simulink model "CommSys_300_Bus_Area2"  (Simulink 8.0)
settings: Solver=ode45  StartTime=0.0  StopTime=85  RelTol=1e-3
libraries: PiccSIM x86
settings Model: Creator=svenda  LastModifiedBy=svenda

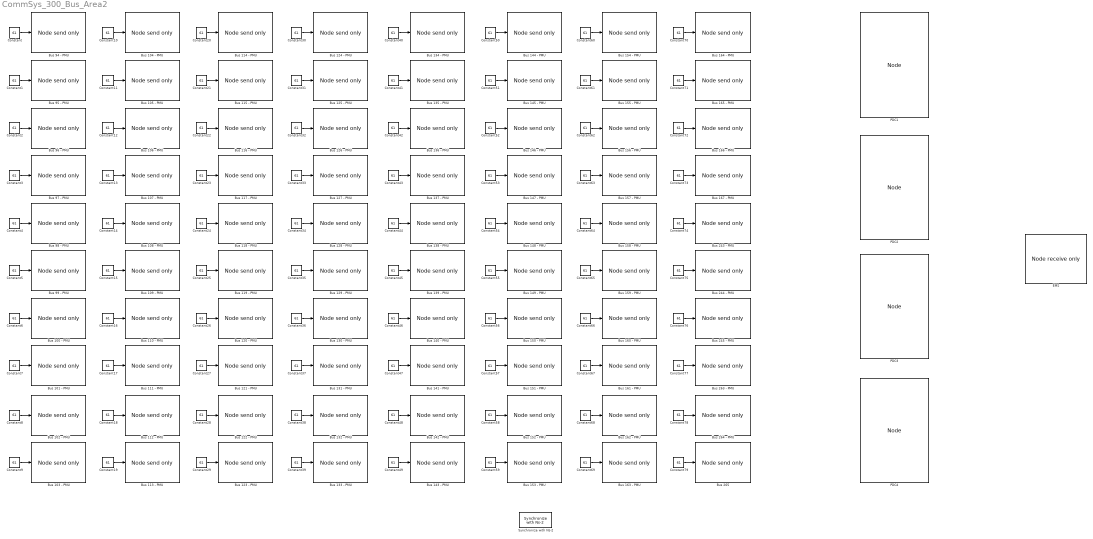
== system CommSys_300_Bus_Area2 ==
  Bus 100 - PMU : PiccSIM/Node send only  ID=6  time_or_seq=Timestamp  sendSchedule=Fixed sampling time  h=0.02  duty_cycle=1  sendEnable=off  pTypesSend=[16]  sendDataStructure={{'double'}}  externalID=off  sendID={[80]}  coordinates=[0, 0]  IP=NS2_IP
  Bus 101 - PMU : PiccSIM/Node send only  ID=7  time_or_seq=Timestamp  sendSchedule=Fixed sampling time  h=0.02  duty_cycle=1  sendEnable=off  pTypesSend=[17]  sendDataStructure={{'double'}}  externalID=off  sendID={[80]}  coordinates=[0, 0]  IP=NS2_IP
  Bus 102 - PMU : PiccSIM/Node send only  ID=8  time_or_seq=Timestamp  sendSchedule=Fixed sampling time  h=0.02  duty_cycle=1  sendEnable=off  pTypesSend=[18]  sendDataStructure={{'double'}}  externalID=off  sendID={[80]}  coordinates=[0, 0]  IP=NS2_IP
  Bus 103 - PMU : PiccSIM/Node send only  ID=9  time_or_seq=Timestamp  sendSchedule=Fixed sampling time  h=0.02  duty_cycle=1  sendEnable=off  pTypesSend=[19]  sendDataStructure={{'double'}}  externalID=off  sendID={[80]}  coordinates=[0, 0]  IP=NS2_IP
  Bus 104 - PMU : PiccSIM/Node send only  ID=10  time_or_seq=Timestamp  sendSchedule=Fixed sampling time  h=0.02  duty_cycle=1  sendEnable=off  pTypesSend=[110]  sendDataStructure={{'double'}}  externalID=off  sendID={[80]}  coordinates=[0, 0]  IP=NS2_IP
  Bus 105 - PMU : PiccSIM/Node send only  ID=11  time_or_seq=Timestamp  sendSchedule=Fixed sampling time  h=0.02  duty_cycle=1  sendEnable=off  pTypesSend=[111]  sendDataStructure={{'double'}}  externalID=off  sendID={[80]}  coordinates=[0, 0]  IP=NS2_IP
  Bus 106 - PMU : PiccSIM/Node send only  ID=12  time_or_seq=Timestamp  sendSchedule=Fixed sampling time  h=0.02  duty_cycle=1  sendEnable=off  pTypesSend=[112]  sendDataStructure={{'double'}}  externalID=off  sendID={[80]}  coordinates=[0, 0]  IP=NS2_IP
  Bus 107 - PMU : PiccSIM/Node send only  ID=13  time_or_seq=Timestamp  sendSchedule=Fixed sampling time  h=0.02  duty_cycle=1  sendEnable=off  pTypesSend=[113]  sendDataStructure={{'double'}}  externalID=off  sendID={[80]}  coordinates=[0, 0]  IP=NS2_IP
  Bus 108 - PMU : PiccSIM/Node send only  ID=14  time_or_seq=Timestamp  sendSchedule=Fixed sampling time  h=0.02  duty_cycle=1  sendEnable=off  pTypesSend=[114]  sendDataStructure={{'double'}}  externalID=off  sendID={[80]}  coordinates=[0, 0]  IP=NS2_IP
  Bus 109 - PMU : PiccSIM/Node send only  ID=15  time_or_seq=Timestamp  sendSchedule=Fixed sampling time  h=0.02  duty_cycle=1  sendEnable=off  pTypesSend=[115]  sendDataStructure={{'double'}}  externalID=off  sendID={[80]}  coordinates=[0, 0]  IP=NS2_IP
  Bus 110 - PMU : PiccSIM/Node send only  ID=16  time_or_seq=Timestamp  sendSchedule=Fixed sampling time  h=0.02  duty_cycle=1  sendEnable=off  pTypesSend=[116]  sendDataStructure={{'double'}}  externalID=off  sendID={[80]}  coordinates=[0, 0]  IP=NS2_IP
  Bus 111 - PMU : PiccSIM/Node send only  ID=17  time_or_seq=Timestamp  sendSchedule=Fixed sampling time  h=0.02  duty_cycle=1  sendEnable=off  pTypesSend=[117]  sendDataStructure={{'double'}}  externalID=off  sendID={[80]}  coordinates=[0, 0]  IP=NS2_IP
  Bus 112 - PMU : PiccSIM/Node send only  ID=18  time_or_seq=Timestamp  sendSchedule=Fixed sampling time  h=0.02  duty_cycle=1  sendEnable=off  pTypesSend=[118]  sendDataStructure={{'double'}}  externalID=off  sendID={[80]}  coordinates=[0, 0]  IP=NS2_IP
  Bus 113 - PMU : PiccSIM/Node send only  ID=19  time_or_seq=Timestamp  sendSchedule=Fixed sampling time  h=0.02  duty_cycle=1  sendEnable=off  pTypesSend=[119]  sendDataStructure={{'double'}}  externalID=off  sendID={[80]}  coordinates=[0, 0]  IP=NS2_IP
  Bus 114 - PMU : PiccSIM/Node send only  ID=20  time_or_seq=Timestamp  sendSchedule=Fixed sampling time  h=0.02  duty_cycle=1  sendEnable=off  pTypesSend=[120]  sendDataStructure={{'double'}}  externalID=off  sendID={[81]}  coordinates=[0, 0]  IP=NS2_IP
  Bus 115 - PMU : PiccSIM/Node send only  ID=21  time_or_seq=Timestamp  sendSchedule=Fixed sampling time  h=0.02  duty_cycle=1  sendEnable=off  pTypesSend=[121]  sendDataStructure={{'double'}}  externalID=off  sendID={[81]}  coordinates=[0, 0]  IP=NS2_IP
  Bus 116 - PMU : PiccSIM/Node send only  ID=22  time_or_seq=Timestamp  sendSchedule=Fixed sampling time  h=0.02  duty_cycle=1  sendEnable=off  pTypesSend=[122]  sendDataStructure={{'double'}}  externalID=off  sendID={[81]}  coordinates=[0, 0]  IP=NS2_IP
  Bus 117 - PMU : PiccSIM/Node send only  ID=23  time_or_seq=Timestamp  sendSchedule=Fixed sampling time  h=0.02  duty_cycle=1  sendEnable=off  pTypesSend=[123]  sendDataStructure={{'double'}}  externalID=off  sendID={[81]}  coordinates=[0, 0]  IP=NS2_IP
  Bus 118 - PMU : PiccSIM/Node send only  ID=24  time_or_seq=Timestamp  sendSchedule=Fixed sampling time  h=0.02  duty_cycle=1  sendEnable=off  pTypesSend=[124]  sendDataStructure={{'double'}}  externalID=off  sendID={[81]}  coordinates=[0, 0]  IP=NS2_IP
  Bus 119 - PMU : PiccSIM/Node send only  ID=25  time_or_seq=Timestamp  sendSchedule=Fixed sampling time  h=0.02  duty_cycle=1  sendEnable=off  pTypesSend=[125]  sendDataStructure={{'double'}}  externalID=off  sendID={[81]}  coordinates=[0, 0]  IP=NS2_IP
  Bus 120 - PMU : PiccSIM/Node send only  ID=26  time_or_seq=Timestamp  sendSchedule=Fixed sampling time  h=0.02  duty_cycle=1  sendEnable=off  pTypesSend=[126]  sendDataStructure={{'double'}}  externalID=off  sendID={[81]}  coordinates=[0, 0]  IP=NS2_IP
  Bus 121 - PMU : PiccSIM/Node send only  ID=27  time_or_seq=Timestamp  sendSchedule=Fixed sampling time  h=0.02  duty_cycle=1  sendEnable=off  pTypesSend=[127]  sendDataStructure={{'double'}}  externalID=off  sendID={[81]}  coordinates=[0, 0]  IP=NS2_IP
  Bus 122 - PMU : PiccSIM/Node send only  ID=28  time_or_seq=Timestamp  sendSchedule=Fixed sampling time  h=0.02  duty_cycle=1  sendEnable=off  pTypesSend=[128]  sendDataStructure={{'double'}}  externalID=off  sendID={[81]}  coordinates=[0, 0]  IP=NS2_IP
  Bus 123 - PMU : PiccSIM/Node send only  ID=29  time_or_seq=Timestamp  sendSchedule=Fixed sampling time  h=0.02  duty_cycle=1  sendEnable=off  pTypesSend=[129]  sendDataStructure={{'double'}}  externalID=off  sendID={[81]}  coordinates=[0, 0]  IP=NS2_IP
  Bus 124 - PMU : PiccSIM/Node send only  ID=30  time_or_seq=Timestamp  sendSchedule=Fixed sampling time  h=0.02  duty_cycle=1  sendEnable=off  pTypesSend=[130]  sendDataStructure={{'double'}}  externalID=off  sendID={[81]}  coordinates=[0, 0]  IP=NS2_IP
  Bus 125 - PMU : PiccSIM/Node send only  ID=31  time_or_seq=Timestamp  sendSchedule=Fixed sampling time  h=0.02  duty_cycle=1  sendEnable=off  pTypesSend=[131]  sendDataStructure={{'double'}}  externalID=off  sendID={[81]}  coordinates=[0, 0]  IP=NS2_IP
  Bus 126 - PMU : PiccSIM/Node send only  ID=32  time_or_seq=Timestamp  sendSchedule=Fixed sampling time  h=0.02  duty_cycle=1  sendEnable=off  pTypesSend=[132]  sendDataStructure={{'double'}}  externalID=off  sendID={[81]}  coordinates=[0, 0]  IP=NS2_IP
  Bus 127 - PMU : PiccSIM/Node send only  ID=33  time_or_seq=Timestamp  sendSchedule=Fixed sampling time  h=0.02  duty_cycle=1  sendEnable=off  pTypesSend=[133]  sendDataStructure={{'double'}}  externalID=off  sendID={[81]}  coordinates=[0, 0]  IP=NS2_IP
  Bus 128 - PMU : PiccSIM/Node send only  ID=34  time_or_seq=Timestamp  sendSchedule=Fixed sampling time  h=0.02  duty_cycle=1  sendEnable=off  pTypesSend=[134]  sendDataStructure={{'double'}}  externalID=off  sendID={[81]}  coordinates=[0, 0]  IP=NS2_IP
  Bus 129 - PMU : PiccSIM/Node send only  ID=35  time_or_seq=Timestamp  sendSchedule=Fixed sampling time  h=0.02  duty_cycle=1  sendEnable=off  pTypesSend=[135]  sendDataStructure={{'double'}}  externalID=off  sendID={[81]}  coordinates=[0, 0]  IP=NS2_IP
  Bus 130 - PMU : PiccSIM/Node send only  ID=36  time_or_seq=Timestamp  sendSchedule=Fixed sampling time  h=0.02  duty_cycle=1  sendEnable=off  pTypesSend=[136]  sendDataStructure={{'double'}}  externalID=off  sendID={[81]}  coordinates=[0, 0]  IP=NS2_IP
  Bus 131 - PMU : PiccSIM/Node send only  ID=37  time_or_seq=Timestamp  sendSchedule=Fixed sampling time  h=0.02  duty_cycle=1  sendEnable=off  pTypesSend=[137]  sendDataStructure={{'double'}}  externalID=off  sendID={[81]}  coordinates=[0, 0]  IP=NS2_IP
  Bus 132 - PMU : PiccSIM/Node send only  ID=38  time_or_seq=Timestamp  sendSchedule=Fixed sampling time  h=0.02  duty_cycle=1  sendEnable=off  pTypesSend=[138]  sendDataStructure={{'double'}}  externalID=off  sendID={[81]}  coordinates=[0, 0]  IP=NS2_IP
  Bus 133 - PMU : PiccSIM/Node send only  ID=39  time_or_seq=Timestamp  sendSchedule=Fixed sampling time  h=0.02  duty_cycle=1  sendEnable=off  pTypesSend=[139]  sendDataStructure={{'double'}}  externalID=off  sendID={[81]}  coordinates=[0, 0]  IP=NS2_IP
  Bus 134 - PMU : PiccSIM/Node send only  ID=40  time_or_seq=Timestamp  sendSchedule=Fixed sampling time  h=0.02  duty_cycle=1  sendEnable=off  pTypesSend=[140]  sendDataStructure={{'double'}}  externalID=off  sendID={[82]}  coordinates=[0, 0]  IP=NS2_IP
  Bus 135 - PMU : PiccSIM/Node send only  ID=41  time_or_seq=Timestamp  sendSchedule=Fixed sampling time  h=0.02  duty_cycle=1  sendEnable=off  pTypesSend=[141]  sendDataStructure={{'double'}}  externalID=off  sendID={[82]}  coordinates=[0, 0]  IP=NS2_IP
  Bus 136 - PMU : PiccSIM/Node send only  ID=42  time_or_seq=Timestamp  sendSchedule=Fixed sampling time  h=0.02  duty_cycle=1  sendEnable=off  pTypesSend=[142]  sendDataStructure={{'double'}}  externalID=off  sendID={[82]}  coordinates=[0, 0]  IP=NS2_IP
  Bus 137 - PMU : PiccSIM/Node send only  ID=43  time_or_seq=Timestamp  sendSchedule=Fixed sampling time  h=0.02  duty_cycle=1  sendEnable=off  pTypesSend=[143]  sendDataStructure={{'double'}}  externalID=off  sendID={[82]}  coordinates=[0, 0]  IP=NS2_IP
  Bus 138 - PMU : PiccSIM/Node send only  ID=44  time_or_seq=Timestamp  sendSchedule=Fixed sampling time  h=0.02  duty_cycle=1  sendEnable=off  pTypesSend=[144]  sendDataStructure={{'double'}}  externalID=off  sendID={[82]}  coordinates=[0, 0]  IP=NS2_IP
  Bus 139 - PMU : PiccSIM/Node send only  ID=45  time_or_seq=Timestamp  sendSchedule=Fixed sampling time  h=0.02  duty_cycle=1  sendEnable=off  pTypesSend=[145]  sendDataStructure={{'double'}}  externalID=off  sendID={[82]}  coordinates=[0, 0]  IP=NS2_IP
  Bus 140 - PMU : PiccSIM/Node send only  ID=46  time_or_seq=Timestamp  sendSchedule=Fixed sampling time  h=0.02  duty_cycle=1  sendEnable=off  pTypesSend=[146]  sendDataStructure={{'double'}}  externalID=off  sendID={[82]}  coordinates=[0, 0]  IP=NS2_IP
  Bus 141 - PMU : PiccSIM/Node send only  ID=47  time_or_seq=Timestamp  sendSchedule=Fixed sampling time  h=0.02  duty_cycle=1  sendEnable=off  pTypesSend=[147]  sendDataStructure={{'double'}}  externalID=off  sendID={[82]}  coordinates=[0, 0]  IP=NS2_IP
  Bus 142 - PMU : PiccSIM/Node send only  ID=48  time_or_seq=Timestamp  sendSchedule=Fixed sampling time  h=0.02  duty_cycle=1  sendEnable=off  pTypesSend=[148]  sendDataStructure={{'double'}}  externalID=off  sendID={[82]}  coordinates=[0, 0]  IP=NS2_IP
  Bus 143 - PMU : PiccSIM/Node send only  ID=49  time_or_seq=Timestamp  sendSchedule=Fixed sampling time  h=0.02  duty_cycle=1  sendEnable=off  pTypesSend=[149]  sendDataStructure={{'double'}}  externalID=off  sendID={[82]}  coordinates=[0, 0]  IP=NS2_IP
  Bus 144 - PMU : PiccSIM/Node send only  ID=50  time_or_seq=Timestamp  sendSchedule=Fixed sampling time  h=0.02  duty_cycle=1  sendEnable=off  pTypesSend=[150]  sendDataStructure={{'double'}}  externalID=off  sendID={[82]}  coordinates=[0, 0]  IP=NS2_IP
  Bus 145 - PMU : PiccSIM/Node send only  ID=51  time_or_seq=Timestamp  sendSchedule=Fixed sampling time  h=0.02  duty_cycle=1  sendEnable=off  pTypesSend=[151]  sendDataStructure={{'double'}}  externalID=off  sendID={[82]}  coordinates=[0, 0]  IP=NS2_IP
  Bus 146 - PMU : PiccSIM/Node send only  ID=52  time_or_seq=Timestamp  sendSchedule=Fixed sampling time  h=0.02  duty_cycle=1  sendEnable=off  pTypesSend=[152]  sendDataStructure={{'double'}}  externalID=off  sendID={[82]}  coordinates=[0, 0]  IP=NS2_IP
  Bus 147 - PMU : PiccSIM/Node send only  ID=53  time_or_seq=Timestamp  sendSchedule=Fixed sampling time  h=0.02  duty_cycle=1  sendEnable=off  pTypesSend=[153]  sendDataStructure={{'double'}}  externalID=off  sendID={[82]}  coordinates=[0, 0]  IP=NS2_IP
  Bus 148 - PMU : PiccSIM/Node send only  ID=54  time_or_seq=Timestamp  sendSchedule=Fixed sampling time  h=0.02  duty_cycle=1  sendEnable=off  pTypesSend=[154]  sendDataStructure={{'double'}}  externalID=off  sendID={[82]}  coordinates=[0, 0]  IP=NS2_IP
  Bus 149 - PMU : PiccSIM/Node send only  ID=55  time_or_seq=Timestamp  sendSchedule=Fixed sampling time  h=0.02  duty_cycle=1  sendEnable=off  pTypesSend=[155]  sendDataStructure={{'double'}}  externalID=off  sendID={[82]}  coordinates=[0, 0]  IP=NS2_IP
  Bus 150 - PMU : PiccSIM/Node send only  ID=56  time_or_seq=Timestamp  sendSchedule=Fixed sampling time  h=0.02  duty_cycle=1  sendEnable=off  pTypesSend=[156]  sendDataStructure={{'double'}}  externalID=off  sendID={[82]}  coordinates=[0, 0]  IP=NS2_IP
  Bus 151 - PMU : PiccSIM/Node send only  ID=57  time_or_seq=Timestamp  sendSchedule=Fixed sampling time  h=0.02  duty_cycle=1  sendEnable=off  pTypesSend=[157]  sendDataStructure={{'double'}}  externalID=off  sendID={[82]}  coordinates=[0, 0]  IP=NS2_IP
  Bus 152 - PMU : PiccSIM/Node send only  ID=58  time_or_seq=Timestamp  sendSchedule=Fixed sampling time  h=0.02  duty_cycle=1  sendEnable=off  pTypesSend=[158]  sendDataStructure={{'double'}}  externalID=off  sendID={[82]}  coordinates=[0, 0]  IP=NS2_IP
  Bus 153 - PMU : PiccSIM/Node send only  ID=59  time_or_seq=Timestamp  sendSchedule=Fixed sampling time  h=0.02  duty_cycle=1  sendEnable=off  pTypesSend=[159]  sendDataStructure={{'double'}}  externalID=off  sendID={[82]}  coordinates=[0, 0]  IP=NS2_IP
  Bus 154 - PMU : PiccSIM/Node send only  ID=60  time_or_seq=Timestamp  sendSchedule=Fixed sampling time  h=0.02  duty_cycle=1  sendEnable=off  pTypesSend=[160]  sendDataStructure={{'double'}}  externalID=off  sendID={[83]}  coordinates=[0, 0]  IP=NS2_IP
  Bus 155 - PMU : PiccSIM/Node send only  ID=61  time_or_seq=Timestamp  sendSchedule=Fixed sampling time  h=0.02  duty_cycle=1  sendEnable=off  pTypesSend=[161]  sendDataStructure={{'double'}}  externalID=off  sendID={[83]}  coordinates=[0, 0]  IP=NS2_IP
  Bus 156 - PMU : PiccSIM/Node send only  ID=62  time_or_seq=Timestamp  sendSchedule=Fixed sampling time  h=0.02  duty_cycle=1  sendEnable=off  pTypesSend=[162]  sendDataStructure={{'double'}}  externalID=off  sendID={[83]}  coordinates=[0, 0]  IP=NS2_IP
  Bus 157 - PMU : PiccSIM/Node send only  ID=63  time_or_seq=Timestamp  sendSchedule=Fixed sampling time  h=0.02  duty_cycle=1  sendEnable=off  pTypesSend=[163]  sendDataStructure={{'double'}}  externalID=off  sendID={[83]}  coordinates=[0, 0]  IP=NS2_IP
  Bus 158 - PMU : PiccSIM/Node send only  ID=64  time_or_seq=Timestamp  sendSchedule=Fixed sampling time  h=0.02  duty_cycle=1  sendEnable=off  pTypesSend=[164]  sendDataStructure={{'double'}}  externalID=off  sendID={[83]}  coordinates=[0, 0]  IP=NS2_IP
  Bus 159 - PMU : PiccSIM/Node send only  ID=65  time_or_seq=Timestamp  sendSchedule=Fixed sampling time  h=0.02  duty_cycle=1  sendEnable=off  pTypesSend=[165]  sendDataStructure={{'double'}}  externalID=off  sendID={[83]}  coordinates=[0, 0]  IP=NS2_IP
  Bus 160 - PMU : PiccSIM/Node send only  ID=66  time_or_seq=Timestamp  sendSchedule=Fixed sampling time  h=0.02  duty_cycle=1  sendEnable=off  pTypesSend=[166]  sendDataStructure={{'double'}}  externalID=off  sendID={[83]}  coordinates=[0, 0]  IP=NS2_IP
  Bus 161 - PMU : PiccSIM/Node send only  ID=67  time_or_seq=Timestamp  sendSchedule=Fixed sampling time  h=0.02  duty_cycle=1  sendEnable=off  pTypesSend=[167]  sendDataStructure={{'double'}}  externalID=off  sendID={[83]}  coordinates=[0, 0]  IP=NS2_IP
  Bus 162 - PMU : PiccSIM/Node send only  ID=68  time_or_seq=Timestamp  sendSchedule=Fixed sampling time  h=0.02  duty_cycle=1  sendEnable=off  pTypesSend=[168]  sendDataStructure={{'double'}}  externalID=off  sendID={[83]}  coordinates=[0, 0]  IP=NS2_IP
  Bus 163 - PMU : PiccSIM/Node send only  ID=69  time_or_seq=Timestamp  sendSchedule=Fixed sampling time  h=0.02  duty_cycle=1  sendEnable=off  pTypesSend=[169]  sendDataStructure={{'double'}}  externalID=off  sendID={[83]}  coordinates=[0, 0]  IP=NS2_IP
  Bus 164 - PMU : PiccSIM/Node send only  ID=70  time_or_seq=Timestamp  sendSchedule=Fixed sampling time  h=0.02  duty_cycle=1  sendEnable=off  pTypesSend=[170]  sendDataStructure={{'double'}}  externalID=off  sendID={[83]}  coordinates=[0, 0]  IP=NS2_IP
  Bus 165 - PMU : PiccSIM/Node send only  ID=71  time_or_seq=Timestamp  sendSchedule=Fixed sampling time  h=0.02  duty_cycle=1  sendEnable=off  pTypesSend=[171]  sendDataStructure={{'double'}}  externalID=off  sendID={[83]}  coordinates=[0, 0]  IP=NS2_IP
  Bus 166 - PMU : PiccSIM/Node send only  ID=72  time_or_seq=Timestamp  sendSchedule=Fixed sampling time  h=0.02  duty_cycle=1  sendEnable=off  pTypesSend=[172]  sendDataStructure={{'double'}}  externalID=off  sendID={[83]}  coordinates=[0, 0]  IP=NS2_IP
  Bus 167 - PMU : PiccSIM/Node send only  ID=73  time_or_seq=Timestamp  sendSchedule=Fixed sampling time  h=0.02  duty_cycle=1  sendEnable=off  pTypesSend=[173]  sendDataStructure={{'double'}}  externalID=off  sendID={[83]}  coordinates=[0, 0]  IP=NS2_IP
  Bus 243 - PMU : PiccSIM/Node send only  ID=74  time_or_seq=Timestamp  sendSchedule=Fixed sampling time  h=0.02  duty_cycle=1  sendEnable=off  pTypesSend=[174]  sendDataStructure={{'double'}}  externalID=off  sendID={[83]}  coordinates=[0, 0]  IP=NS2_IP
  Bus 244 - PMU : PiccSIM/Node send only  ID=75  time_or_seq=Timestamp  sendSchedule=Fixed sampling time  h=0.02  duty_cycle=1  sendEnable=off  pTypesSend=[175]  sendDataStructure={{'double'}}  externalID=off  sendID={[83]}  coordinates=[0, 0]  IP=NS2_IP
  Bus 245 - PMU : PiccSIM/Node send only  ID=76  time_or_seq=Timestamp  sendSchedule=Fixed sampling time  h=0.02  duty_cycle=1  sendEnable=off  pTypesSend=[176]  sendDataStructure={{'double'}}  externalID=off  sendID={[83]}  coordinates=[0, 0]  IP=NS2_IP
  Bus 263 - PMU : PiccSIM/Node send only  ID=77  time_or_seq=Timestamp  sendSchedule=Fixed sampling time  h=0.02  duty_cycle=1  sendEnable=off  pTypesSend=[177]  sendDataStructure={{'double'}}  externalID=off  sendID={[83]}  coordinates=[0, 0]  IP=NS2_IP
  "Bus 264 - PMU " : PiccSIM/Node send only  ID=78  time_or_seq=Timestamp  sendSchedule=Fixed sampling time  h=0.02  duty_cycle=1  sendEnable=off  pTypesSend=[178]  sendDataStructure={{'double'}}  externalID=off  sendID={[83]}  coordinates=[0, 0]  IP=NS2_IP
  Bus 265 : PiccSIM/Node send only  ID=79  time_or_seq=Timestamp  sendSchedule=Fixed sampling time  h=0.02  duty_cycle=1  sendEnable=off  pTypesSend=[179]  sendDataStructure={{'double'}}  externalID=off  sendID={[83]}  coordinates=[0, 0]  IP=NS2_IP
  Bus 94 - PMU : PiccSIM/Node send only  ID=0  time_or_seq=Timestamp  sendSchedule=Fixed sampling time  h=0.02  duty_cycle=1  sendEnable=off  pTypesSend=[10]  sendDataStructure={{'double'}}  externalID=off  sendID={[80]}  coordinates=[0, 0]  IP=NS2_IP
  Bus 95 - PMU : PiccSIM/Node send only  ID=1  time_or_seq=Timestamp  sendSchedule=Fixed sampling time  h=0.02  duty_cycle=1  sendEnable=off  pTypesSend=[11]  sendDataStructure={{'double'}}  externalID=off  sendID={[80]}  coordinates=[0, 0]  IP=NS2_IP
  Bus 96 - PMU : PiccSIM/Node send only  ID=2  time_or_seq=Timestamp  sendSchedule=Fixed sampling time  h=0.02  duty_cycle=1  sendEnable=off  pTypesSend=[12]  sendDataStructure={{'double'}}  externalID=off  sendID={[80]}  coordinates=[0, 0]  IP=NS2_IP
  Bus 97 - PMU : PiccSIM/Node send only  ID=3  time_or_seq=Timestamp  sendSchedule=Fixed sampling time  h=0.02  duty_cycle=1  sendEnable=off  pTypesSend=[13]  sendDataStructure={{'double'}}  externalID=off  sendID={[80]}  coordinates=[0, 0]  IP=NS2_IP
  Bus 98 - PMU : PiccSIM/Node send only  ID=4  time_or_seq=Timestamp  sendSchedule=Fixed sampling time  h=0.02  duty_cycle=1  sendEnable=off  pTypesSend=[14]  sendDataStructure={{'double'}}  externalID=off  sendID={[80]}  coordinates=[0, 0]  IP=NS2_IP
  Bus 99 - PMU : PiccSIM/Node send only  ID=5  time_or_seq=Timestamp  sendSchedule=Fixed sampling time  h=0.02  duty_cycle=1  sendEnable=off  pTypesSend=[15]  sendDataStructure={{'double'}}  externalID=off  sendID={[80]}  coordinates=[0, 0]  IP=NS2_IP
  Constant{,1..79} (80 alike) : Constant  Value=61
  EMS : PiccSIM/Node receive only  ID=84  pTypes=[180, 181, 182, 183]  receiveDataLengths={{[1]}, {[1]}, {[1]}, {[1]}}  receiveDataStructure={{'double'}, {'double'}, {'double'}, {'double'}}  recFrom={[80], [81], [82], [83]}  coordinates=[0, 0]  IP=NS2_IP
  PDC1 : PiccSIM/Node  ID=80  time_or_seq=Timestamp  sendSchedule=Fixed sampling time  h=0.02  duty_cycle=1  sendEnable=off  pTypesSend=[180]  sendDataStructure={{'double'}}  externalID=off  sendID={[84]}  pTypes=[10, 11, 12, 13, 14, 15, 16, 17, 18, 19, 110, 111, 112, 113, 114, 115, 116, 117, 118, 119]  receiveDataLengths={{[1]}, {[1]}, {[1]}, {[1]}, {[1]}, {[1]}, {[1]}, {[1]}, {[1]}, {[1]},{[1]}, {[1]}, {[1]}, {[1]}, {[1]}, {[1]}, {[1]}, {[1]}, {[1]}, {[1]}}  receiveDataStructure={{'double'}, {'double'}, {'double'}, {'double'}, {'double'}, {'double'}, {'double'}, {'double'}, {'double'}, {'double'}, {'double'}, {'double'}, {'double'}, {'double'}, {'double'}, {'double'}, {'double'}, {'double'}, {'double'}, {'double'}}  recFrom={[0], [1], [2], [3], [4], [5], [6], [7], [8], [9], [10], [11], [12], [13], [14], [15], [16], [17], [18], [19]}  coordinates=[0, 0]  IP=NS2_IP
  PDC2 : PiccSIM/Node  ID=81  time_or_seq=Timestamp  sendSchedule=Fixed sampling time  h=0.02  duty_cycle=1  sendEnable=off  pTypesSend=[181]  sendDataStructure={{'double'}}  externalID=off  sendID={[84]}  pTypes=[120, 121, 122, 123, 124, 125, 126, 127, 128, 129, 130, 131, 132, 133, 134, 135, 136, 137, 138, 139]  receiveDataLengths={{[1]}, {[1]}, {[1]}, {[1]}, {[1]}, {[1]}, {[1]}, {[1]}, {[1]}, {[1]},{[1]}, {[1]}, {[1]}, {[1]}, {[1]}, {[1]}, {[1]}, {[1]}, {[1]}, {[1]}}  receiveDataStructure={{'double'}, {'double'}, {'double'}, {'double'}, {'double'}, {'double'}, {'double'}, {'double'}, {'double'}, {'double'}, {'double'}, {'double'}, {'double'}, {'double'}, {'double'}, {'double'}, {'double'}, {'double'}, {'double'}, {'double'}}  recFrom={[20], [21], [22], [23], [24], [25], [26], [27], [28], [29], [30], [31], [32], [33], [34], [35], [36], [37], [38], [39]}  coordinates=[0, 0]  IP=NS2_IP
  PDC3 : PiccSIM/Node  ID=82  time_or_seq=Timestamp  sendSchedule=Fixed sampling time  h=0.02  duty_cycle=1  sendEnable=off  pTypesSend=[182]  sendDataStructure={{'double'}}  externalID=off  sendID={[84]}  pTypes=[140, 141, 142, 143, 144, 145, 146, 147, 148, 149, 150, 151, 152, 153, 154, 155, 156, 157, 158, 159]  receiveDataLengths={{[1]}, {[1]}, {[1]}, {[1]}, {[1]}, {[1]}, {[1]}, {[1]}, {[1]}, {[1]},{[1]}, {[1]}, {[1]}, {[1]}, {[1]}, {[1]}, {[1]}, {[1]}, {[1]}, {[1]}}  receiveDataStructure={{'double'}, {'double'}, {'double'}, {'double'}, {'double'}, {'double'}, {'double'}, {'double'}, {'double'}, {'double'}, {'double'}, {'double'}, {'double'}, {'double'}, {'double'}, {'double'}, {'double'}, {'double'}, {'double'}, {'double'}}  recFrom={[40], [41], [42], [43], [44], [45], [46], [47], [48], [49], [50], [51], [52], [53], [54], [55], [56], [57], [58], [59]}  coordinates=[0, 0]  IP=NS2_IP
  PDC4 : PiccSIM/Node  ID=83  time_or_seq=Timestamp  sendSchedule=Fixed sampling time  h=0.02  duty_cycle=1  sendEnable=off  pTypesSend=[183]  sendDataStructure={{'double'}}  externalID=off  sendID={[84]}  pTypes=[160, 161, 162, 163, 164, 165, 166, 167, 168, 169, 170, 171, 172, 173, 174, 175, 176, 177, 178, 179]  receiveDataLengths={{[1]}, {[1]}, {[1]}, {[1]}, {[1]}, {[1]}, {[1]}, {[1]}, {[1]}, {[1]},{[1]}, {[1]}, {[1]}, {[1]}, {[1]}, {[1]}, {[1]}, {[1]}, {[1]}, {[1]}}  receiveDataStructure={{'double'}, {'double'}, {'double'}, {'double'}, {'double'}, {'double'}, {'double'}, {'double'}, {'double'}, {'double'}, {'double'}, {'double'}, {'double'}, {'double'}, {'double'}, {'double'}, {'double'}, {'double'}, {'double'}, {'double'}}  recFrom={[60], [61], [62], [63], [64], [65], [66], [67], [68], [69], [70], [71], [72], [73], [74], [75], [76], [77], [78], [79]}  coordinates=[0, 0]  IP=NS2_IP
  Synchronize with Ns-2 : PiccSIM/Synchronize with Ns-2  Priority=100000  c=1  port=23201  IP=NS2_IP
  wires:
  Constant/1 -> Bus 94 - PMU/1
  Constant1/1 -> Bus 95 - PMU/1
  Constant2/1 -> Bus 96 - PMU/1
  Constant3/1 -> Bus 97 - PMU/1
  Constant4/1 -> Bus 98 - PMU/1
  Constant5/1 -> Bus 99 - PMU/1
  Constant6/1 -> Bus 100 - PMU/1
  Constant7/1 -> Bus 101 - PMU/1
  Constant8/1 -> Bus 102 - PMU/1
  Constant9/1 -> Bus 103 - PMU/1
  Constant10/1 -> Bus 104 - PMU/1
  Constant11/1 -> Bus 105 - PMU/1
  Constant12/1 -> Bus 106 - PMU/1
  Constant13/1 -> Bus 107 - PMU/1
  Constant14/1 -> Bus 108 - PMU/1
  Constant15/1 -> Bus 109 - PMU/1
  Constant16/1 -> Bus 110 - PMU/1
  Constant17/1 -> Bus 111 - PMU/1
  Constant18/1 -> Bus 112 - PMU/1
  Constant19/1 -> Bus 113 - PMU/1
  Constant20/1 -> Bus 114 - PMU/1
  Constant21/1 -> Bus 115 - PMU/1
  Constant22/1 -> Bus 116 - PMU/1
  Constant23/1 -> Bus 117 - PMU/1
  Constant24/1 -> Bus 118 - PMU/1
  Constant25/1 -> Bus 119 - PMU/1
  Constant26/1 -> Bus 120 - PMU/1
  Constant27/1 -> Bus 121 - PMU/1
  Constant28/1 -> Bus 122 - PMU/1
  Constant29/1 -> Bus 123 - PMU/1
  Constant30/1 -> Bus 124 - PMU/1
  Constant31/1 -> Bus 125 - PMU/1
  Constant32/1 -> Bus 126 - PMU/1
  Constant33/1 -> Bus 127 - PMU/1
  Constant34/1 -> Bus 128 - PMU/1
  Constant35/1 -> Bus 129 - PMU/1
  Constant36/1 -> Bus 130 - PMU/1
  Constant37/1 -> Bus 131 - PMU/1
  Constant38/1 -> Bus 132 - PMU/1
  Constant39/1 -> Bus 133 - PMU/1
  Constant40/1 -> Bus 134 - PMU/1
  Constant41/1 -> Bus 135 - PMU/1
  Constant42/1 -> Bus 136 - PMU/1
  Constant43/1 -> Bus 137 - PMU/1
  Constant44/1 -> Bus 138 - PMU/1
  Constant45/1 -> Bus 139 - PMU/1
  Constant46/1 -> Bus 140 - PMU/1
  Constant47/1 -> Bus 141 - PMU/1
  Constant48/1 -> Bus 142 - PMU/1
  Constant49/1 -> Bus 143 - PMU/1
  Constant50/1 -> Bus 144 - PMU/1
  Constant51/1 -> Bus 145 - PMU/1
  Constant52/1 -> Bus 146 - PMU/1
  Constant53/1 -> Bus 147 - PMU/1
  Constant54/1 -> Bus 148 - PMU/1
  Constant55/1 -> Bus 149 - PMU/1
  Constant56/1 -> Bus 150 - PMU/1
  Constant57/1 -> Bus 151 - PMU/1
  Constant58/1 -> Bus 152 - PMU/1
  Constant59/1 -> Bus 153 - PMU/1
  Constant60/1 -> Bus 154 - PMU/1
  Constant61/1 -> Bus 155 - PMU/1
  Constant62/1 -> Bus 156 - PMU/1
  Constant63/1 -> Bus 157 - PMU/1
  Constant64/1 -> Bus 158 - PMU/1
  Constant65/1 -> Bus 159 - PMU/1
  Constant66/1 -> Bus 160 - PMU/1
  Constant67/1 -> Bus 161 - PMU/1
  Constant68/1 -> Bus 162 - PMU/1
  Constant69/1 -> Bus 163 - PMU/1
  Constant70/1 -> Bus 164 - PMU/1
  Constant71/1 -> Bus 165 - PMU/1
  Constant72/1 -> Bus 166 - PMU/1
  Constant73/1 -> Bus 167 - PMU/1
  Constant74/1 -> Bus 243 - PMU/1
  Constant75/1 -> Bus 244 - PMU/1
  Constant76/1 -> Bus 245 - PMU/1
  Constant77/1 -> Bus 263 - PMU/1
  Constant78/1 -> "Bus 264 - PMU "/1
  Constant79/1 -> Bus 265/1
